simulink model "model"  (R2024b)
settings: Solver=VariableStepAuto  StartTime=0.0  StopTime=32  RelTol=1e-3
values from neighbouring files (symbols this model uses):
  b = 20    [main.m]
  br = 5    [main.m]
  L = 1    [main.m]
  w = 0.6    [main.m]
libraries: shared6dof x1, robotcorelib x1, simulink_extras x1, slpidlib x1, uavutilslib x1, uavalgslib x1
settings Model: Creator=awolek  LastModifiedBy=alexn
settings SolverCC: ZeroCrossAlgorithm=Adaptive
settings DebuggingCC: IgnoredZcDiagnostic=none
settings RTWCC: GPUComputeCapability=3.5

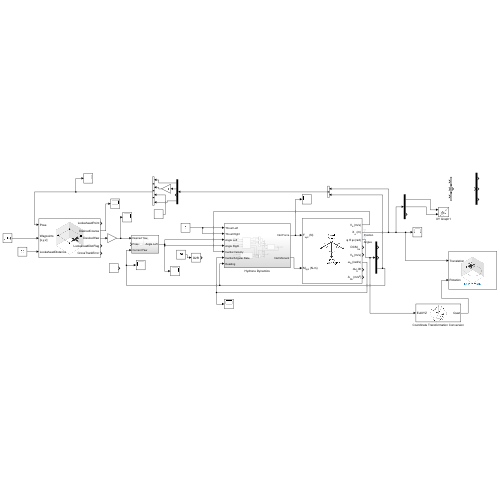
[thumbnail: Simulink's stored preview of the top-level diagram]
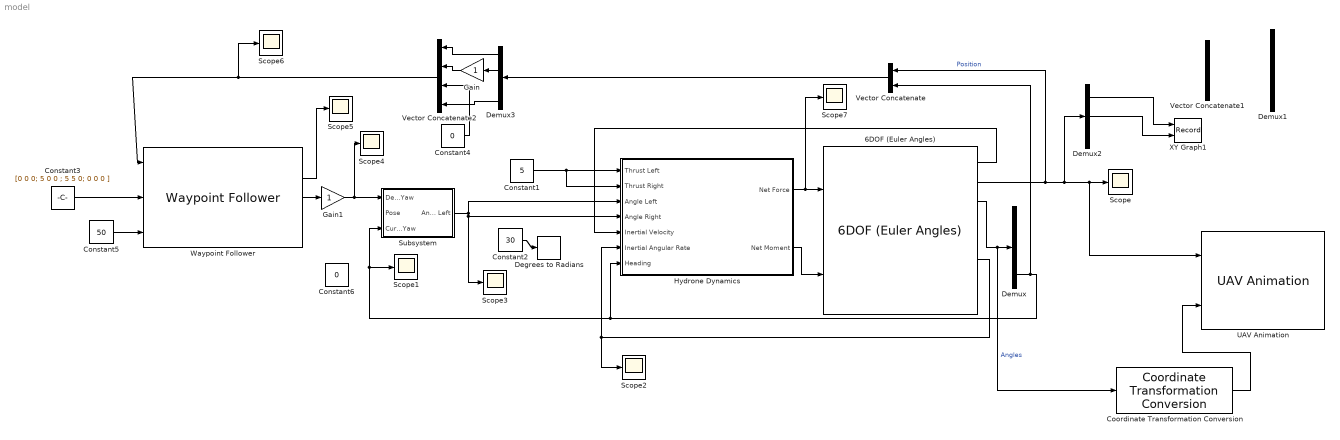
== system model ==
  6DOF (Euler Angles) : shared6dof/6DOF (Euler Angles)  units=Metric (MKS)  mtype=Fixed  rep=Euler Angles  xme_0=[0 0 0]  Vm_0=[0 0 0]  eul_0=[0 0 0]  pm_0=[0 0 0]  mass_0=m  mass_e=0.5  mass_f=2.0  inertia=I  inertia_e=eye(3)  inertia_f=2*eye(3)  k_quat=1.0  vre_flag=on  abi_flag=off  aMode=0  xme_statename=''  Vm_statename=''  eul_statename=''  quat_statename=''  pm_statename=''  mass_statename=''
  Constant1 : Constant  Value=5
  Constant2 : Constant  Value=30
  Constant3 : Constant  Value=[0 0 0; 5 0 0 ; 5 5 0; 0 0 0 ]
  Constant4 : Constant  Value=0
  Constant5 : Constant  Value=50
  Constant6 : Constant  Value=0
  Coordinate Transformation Conversion : robotcorelib/Coordinate Transformation Conversion  InputRepresentation=Euler Angles  InputEulerSequence=XYZ  ShowTrVecInputPort=on  OutputRepresentation=Quaternion  OutputEulerSequence=ZYX  ShowTrVecOutputPort=on  SimulateUsing=Interpreted execution
  Degrees to Radians : simulink_extras/Transformations/Degrees to Radians
  Demux : Demux  Outputs=3
  Demux1 : Demux  Outputs=3
  Demux2 : Demux  Outputs=3
  Demux3 : Demux
  Gain : Gain
  Gain1 : Gain
  Hydrone Dynamics : Subsystem
  Scope{,1..7} (8 alike) : Scope
  Subsystem : Subsystem
  UAV Animation : uavutilslib/UAV Animation  NumUAV=1  DynamicUAVConfig=off  UAVType=Multirotor  UAVSize=1  UAVColor=[1 0 0]  UAVTrajectoryAlpha=1  InertialZDirection=Down  RotationFormat=Quaternion  DrawMarkers=off  SampleTime=-1
  Vector Concatenate : Concatenate
  Vector Concatenate1 : Concatenate  NumInputs=3
  Vector Concatenate2 : Concatenate  NumInputs=4
  Waypoint Follower : uavalgslib/Waypoint Follower  UAVType=fixed-wing  StartFrom=first  TransitionRadiusSource=internal  TransitionRadius=2  MinLookaheadDistance=0.1  HoverAtLastWaypoint=off  YawInput=off  ShowCrossTrackErrorOutput=on  ShowStatusOutput=off  SimulateUsing=Interpreted execution
  XY Graph1 : Record  FileSettingsInternal="{\"entries\":[{\"content\":{\"excelSettings\":{\"content\":{},\"type\":\"Streamout.ExcelSettings\"}},\"type\":\"Streamout.FileSettingStorage\",\"uuid\":\"\"}],\"packageUris\":[\"http:\\/\\/schema.mathworks.com\\/mf0\\/streamout_blocks\\/R2020a\"],\"version\":\"1.0\"}"  Layout=[1 1]  SignalsInternal="{\"entries\":[{\"content\":{\"signals\":[{\"content\":{\"blockPath\":[],\"dimensions\":[1],\"domain\":\"\",\"lineColor\":\"#a2142f\",\"plots\":[ 1 ],\"port\":1,\"sid\":[\"\"],\"signalID\":1,\"signalName\":\"Demux2:1\"},\"type\":\"RecordBlkView.Signal\",\"uuid\":\"\"},{\"content\":{\"blockPath\":[],\"dimensions\":[1],\"domain\":\"\",\"lineColor\":\"#139fff\",\"plots\":[ 1 ],\"port\":2,\"sid\":[\"\"],\"signalID\":2,\"signalName\":\"Demux2:2\"},\"type\":\"RecordBlkView.Signal\",\"uuid\":\"\"}]},\"type\":\"RecordBlkView.InputSignals\",\"uuid\":\"\"}],\"packageUris\":[\"http:\\/\\/schema.mathworks.com\\/mf0\\/streamout_blocks\\/R2020a\"],\"version\":\"1.0\"}"  VisualizationBindings="{\"xyplotplugin\":{\"info\":[{\"series\":[{\"bindingParametersList\":[{\"parameter\":\"X-Axis\",\"signalID\":1,\"signalName\":\"Demux2:1\"},{\"parameter\":\"Y-Axis\",\"signalID\":2,\"signalName\":\"Demux2:2\"},{\"parameter\":\"X-Axis\",\"signalID\":1,\"signalName\":\"Demux2:1\"},{\"parameter\":\"Y-Axis\",\"signalID\":2,\"signalName\":\"Demux2:2\"}],\"seriesID\":0}],\"subplotID\":1}]}}"  CompatibilityTag=XY
  wires:
  Demux/3 -> Vector Concatenate/2, Scope1/1, Subsystem/3(Current Yaw), Hydrone Dynamics/7(Heading)
  Constant2/1 -> Degrees to Radians/1
  Constant1/1 -> Hydrone Dynamics/2(Thrust Right), Hydrone Dynamics/1(Thrust Left)
  6DOF (Euler Angles)/2 -> Vector Concatenate/1, Demux2/1, UAV Animation/1, Scope/1  "Position"
  Hydrone Dynamics/1(Net Force) -> Scope7/1, 6DOF (Euler Angles)/1
  Hydrone Dynamics/2(Net Moment) -> 6DOF (Euler Angles)/2
  6DOF (Euler Angles)/1 -> Hydrone Dynamics/5(Inertial Velocity)
  6DOF (Euler Angles)/3 -> Coordinate Transformation Conversion/1, Demux/1  "Angles"
  6DOF (Euler Angles)/6 -> Hydrone Dynamics/6(Inertial Angular Rate), Scope2/1
  Constant3/1 -> Waypoint Follower/2
  Vector Concatenate/1 -> Demux3/1
  Waypoint Follower/3 -> Gain1/1
  Subsystem/1(Angle Left) -> Hydrone Dynamics/4(Angle Right), Scope3/1, Hydrone Dynamics/3(Angle Left)
  Waypoint Follower/2 -> Scope5/1
  Demux3/1 -> Vector Concatenate2/1
  Demux3/4 -> Vector Concatenate2/4
  Constant4/1 -> Vector Concatenate2/3
  Vector Concatenate2/1 -> Scope6/1, Waypoint Follower/1
  Constant5/1 -> Waypoint Follower/3
  Demux2/1 -> XY Graph1/1
  Demux2/2 -> XY Graph1/2
  Demux3/2 -> Gain/1
  Gain/1 -> Vector Concatenate2/2
  Gain1/1 -> Scope4/1, Subsystem/1(Desired Yaw)
  Coordinate Transformation Conversion/1 -> UAV Animation/2

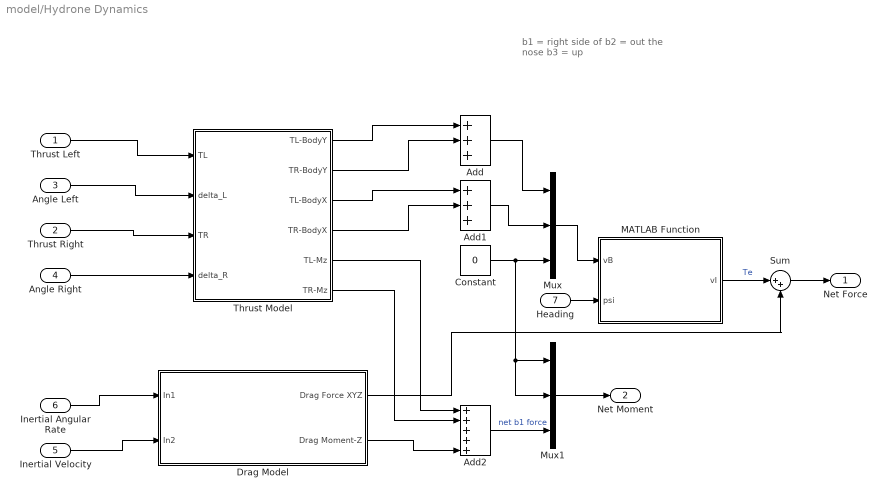
== system model/Hydrone Dynamics ==
  note: b1 = right side of
      | b2 = out the nose
      | b3 = up
  Thrust Left : Inport
  Thrust Right : Inport  Port=2
  Angle Left : Inport  Port=3
  Angle Right : Inport  Port=4
  Inertial Velocity : Inport  Port=5
  Inertial Angular Rate : Inport  Port=6
  Heading : Inport  Port=7
  Add : Sum  Inputs=+++
  Add1 : Sum  Inputs=+++
  Add2 : Sum  Inputs=+++++
  Constant : Constant  Value=0
  Drag Model : Subsystem
  MATLAB Function : MATLAB Function  TreatAsAtomicUnit=on
  Mux : Mux  Inputs=3
  Mux1 : Mux  Inputs=3
  Sum : Sum  Inputs=|++
  Thrust Model : Subsystem
  Net Force : Outport
  Net Moment : Outport  Port=2
  wires:
  Sum/1 -> Net Force/1
  Heading/1 -> MATLAB Function/2(psi)
  Add2/1 -> Mux1/3  "net b1 force"
  Constant/1 -> Mux1/2, Mux1/1, Mux/3
  Drag Model/2(Drag Moment-Z) -> Add2/5
  Mux1/1 -> Net Moment/1
  Drag Model/1(Drag Force XYZ) -> Sum/2
  Thrust Right/1 -> Thrust Model/3(TR)
  Angle Right/1 -> Thrust Model/4(delta_R)
  Add1/1 -> Mux/2
  Inertial Angular Rate/1 -> Drag Model/1(In1)
  MATLAB Function/1(vI) -> Sum/1  "Te"
  Mux/1 -> MATLAB Function/1(vB)
  Thrust Model/6(TR-Mz) -> Add2/2
  Add/1 -> Mux/1
  Thrust Model/1(TL-BodyY) -> Add/1
  Thrust Model/2(TR-BodyY) -> Add/2
  Inertial Velocity/1 -> Drag Model/2(In2)
  Thrust Model/3(TL-BodyX) -> Add1/1
  Angle Left/1 -> Thrust Model/2(delta_L)
  Thrust Model/5(TL-Mz) -> Add2/1
  Thrust Left/1 -> Thrust Model/1(TL)
  Thrust Model/4(TR-BodyX) -> Add1/2

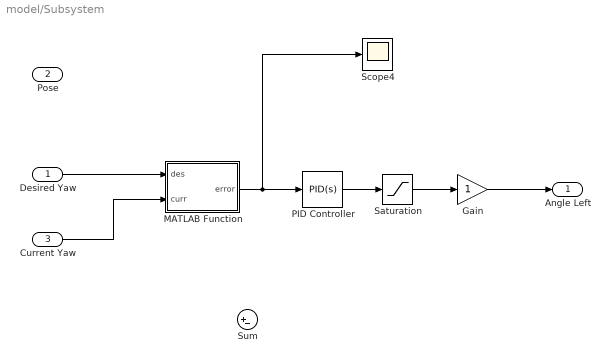
== system model/Subsystem ==
  Desired Yaw : Inport
  Pose : Inport  Port=2
  Current Yaw : Inport  Port=3
  Gain : Gain
  MATLAB Function : MATLAB Function  TreatAsAtomicUnit=on
  PID Controller : slpidlib/PID Controller  Controller=PID  Form=Parallel  TimeDomain=Continuous-time  UseExternalTs=off  SampleTime=-1  IntegratorMethod=Forward Euler  FilterMethod=Forward Euler  ControllerParametersSource=internal  P=1  I=0  UseKiTs=off  D=0  UseExternalDerivativeSource=off  N=100  UseFilter=on  TunerSelectOption=Transfer Function Based (PID Tuner App)  InitialConditionSource=internal  InitialConditionForIntegrator=0  InitialConditionForFilter=0  DifferentiatorICPrevScaledInput=0  ExternalReset=none  TrackingMode=off  Kt=1  LimitOutput=off  SatLimitsSource=internal  UpperSaturationLimit=inf  LowerSaturationLimit=-inf  LinearizeAsGain=on  AntiWindupMode=none  Kb=1  LimitIntegrator=off  UpperIntegratorSaturationLimit=inf  LowerIntegratorSaturationLimit=-inf  POutMin=[]  POutMax=[]  IOutMin=[]  IOutMax=[]  DOutMin=[]  DOutMax=[]  NOutMin=[]  NOutMax=[]  SumOutMin=[]  SumOutMax=[]  SaturationOutMin=[]  SaturationOutMax=[]  PParamMin=[]  PParamMax=[]  IParamMin=[]  IParamMax=[]  DParamMin=[]  DParamMax=[]  NParamMin=[]  NParamMax=[]  KbParamMin=[]  KbParamMax=[]  KtParamMin=[]  KtParamMax=[]  KbOutMin=[]  KbOutMax=[]  KtOutMin=[]  KtOutMax=[]  IntegratorOutMin=[]  IntegratorOutMax=[]  FilterOutMin=[]  FilterOutMax=[]  SumI1OutMin=[]  SumI1OutMax=[]  SumI2OutMin=[]  SumI2OutMax=[]  SumI3OutMin=[]  SumI3OutMax=[]  SumI4OutMin=[]  SumI4OutMax=[]  SumDOutMin=[]  SumDOutMax=[]  DifferentiatorOutMin=[]  DifferentiatorOutMax=[]  FilterDiffOutCoefMin=[]  FilterDiffOutCoefMax=[]  ReciprocalOutMin=[]  ReciprocalOutMax=[]  SumDenOutMin=[]  SumDenOutMax=[]  SumNumOutMin=[]  SumNumOutMax=[]  DivideOutMin=[]  DivideOutMax=[]  UdiffTsProdOutMin=[]  UdiffTsProdOutMax=[]  NTsProdOutMin=[]  NTsProdOutMax=[]  UintegralTsProdOutMin=[]  UintegralTsProdOutMax=[]  UngainTsProdOutMin=[]  UngainTsProdOutMax=[]  ClampingZeroOutDataTypeStr=Inherit: Inherit via back propagation  ClampingZeroOutMin=[]  ClampingZeroOutMax=[]  FilterDenConstantOutDataTypeStr=Inherit: Inherit via back propagation  FilterDenConstantOutMin=[]  FilterDenConstantOutMax=[]  PCopyOutDataTypeStr=Inherit: Inherit via back propagation  PCopyOutMin=[]  PCopyOutMax=[]  NCopyOutDataTypeStr=Inherit: Inherit via back propagation  NCopyOutMin=[]  NCopyOutMax=[]  IntegratorContinuousStateAttributes=''  IntegratorStateMustResolveToSignalObject=off  IntegratorRTWStateStorageClass=Auto  FilterContinuousStateAttributes=''  FilterStateMustResolveToSignalObject=off  FilterRTWStateStorageClass=Auto  ParallelPVariant=InternalParameters  IdealPVariant=Disabled  IVariant=InternalParameters  DVariant=InternalParameters  IntegratorVariant=Continuous  SatVariant=Disabled  AWVariant=Passthrough  PCopyVariant=Disabled  TRVariant=Disabled  FdbkBlocksVariant=Forward  IdealPFdbkVariant=Disabled  SatFdbkVariant=Disabled  DerivativeFilterVariant=ContFilter  NVariant=InternalParameters  NCopyVariant=Disabled  FilterICVariant=InternalICsFilter  IntegratorICVariant=InternalICs  ExternalResetVariant=Disabled  TRSumVariant=Passthrough  SumFdbkVariant=Disabled  SumVariant=Sum_PID  TsampFilterVariant=InternalTs  TsampNgainVariant=Passthrough  TsampIntegralVariant=Disabled_SignalSpec  ExternalSaturationOutDataTypeStr=Inherit: Same as second input  DerivativeSourceVariant=ErrorSignal  PreIntVariant=InternalPreInt
  Saturation : Saturate  UpperLimit=.78  LowerLimit=-.78  LinearizeAsGain=off  ZeroCross=off
  Scope4 : Scope
  Sum : Sum  Inputs=|+-
  Angle Left : Outport
  wires:
  Desired Yaw/1 -> MATLAB Function/1(des)
  PID Controller/1 -> Saturation/1
  Saturation/1 -> Gain/1
  Gain/1 -> Angle Left/1
  Current Yaw/1 -> MATLAB Function/2(curr)
  MATLAB Function/1(error) -> Scope4/1, PID Controller/1

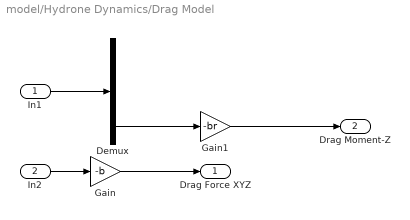
== system model/Hydrone Dynamics/Drag Model ==
  In1 : Inport
  In2 : Inport  Port=2
  Demux : Demux  Outputs=3
  Gain : Gain  Gain=-b
  Gain1 : Gain  Gain=-br
  Drag Force XYZ : Outport
  Drag Moment-Z : Outport  Port=2
  wires:
  Gain1/1 -> Drag Moment-Z/1
  Gain/1 -> Drag Force XYZ/1
  In2/1 -> Gain/1
  In1/1 -> Demux/1
  Demux/3 -> Gain1/1

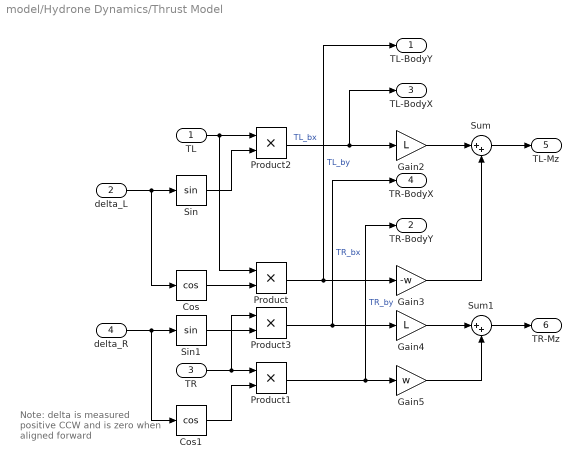
== system model/Hydrone Dynamics/Thrust Model ==
  note: Note: delta is measured
      | positive CCW and is
      | zero when aligned
      | forward
  TL : Inport
  delta_L : Inport  Port=2
  TR : Inport  Port=3
  delta_R : Inport  Port=4
  Cos : Trigonometry  Operator=cos
  Cos1 : Trigonometry  Operator=cos
  Gain2 : Gain  Gain=L
  Gain3 : Gain  Gain=-w
  Gain4 : Gain  Gain=L
  Gain5 : Gain  Gain=w
  Product{,1..3} (4 alike) : Product
  Sin : Trigonometry
  Sin1 : Trigonometry
  Sum : Sum  Inputs=|++
  Sum1 : Sum  Inputs=|++
  TL-BodyY : Outport
  TR-BodyY : Outport  Port=2
  TL-BodyX : Outport  Port=3
  TR-BodyX : Outport  Port=4
  TL-Mz : Outport  Port=5
  TR-Mz : Outport  Port=6
  wires:
  Sum/1 -> TL-Mz/1
  Gain5/1 -> Sum1/2
  Gain4/1 -> Sum1/1
  delta_L/1 -> Cos/1, Sin/1
  Cos1/1 -> Product1/2
  delta_R/1 -> Cos1/1, Sin1/1
  TR/1 -> Product3/1, Product1/1
  TL/1 -> Product/1, Product2/1
  Sin1/1 -> Product3/2
  Sin/1 -> Product2/2
  Sum1/1 -> TR-Mz/1
  Gain3/1 -> Sum/2
  Product/1 -> TL-BodyY/1, Gain3/1  "TL_by"
  Cos/1 -> Product/2
  Product2/1 -> TL-BodyX/1, Gain2/1  "TL_bx"
  Product3/1 -> Gain4/1, TR-BodyX/1  "TR_bx"
  Product1/1 -> TR-BodyY/1, Gain5/1  "TR_by"
  Gain2/1 -> Sum/1

== matlab function model/Hydrone Dynamics/MATLAB Function ==
  data: vB input; vI output; psi input
function vI = R_BtoI(vB, psi)

R_BtoI = [cos(psi) sin(psi) 0;
         sin(psi) -cos(psi) 0;
         0         0        1];
vI = R_BtoI*vB;

== matlab function model/Subsystem/MATLAB Function ==
  data: des input; error output; curr input
function error = fcn(des,curr)

error = atan2(sin(des-curr),cos(des-curr));

% if des <  (curr + pi/2) || des > (curr - pi/2) 
%     error=abs(error);
% else
%     error=abs(error)*-1;
% end
